simulink subsystem "Tire_Force"  (R2021b)
settings: Solver=VariableStepAuto  StartTime=0.0  StopTime=10.0  RelTol=1e-3
values from neighbouring files (symbols this model uses):
  afx_f = [1.736519934348130,-2.903281841026900e-04,2.651682004580759,7.000047010028531e+04,3.270011055825476e+03,-0.001252141095807,1.596836353939939]    [OneWheelModel_test1.m]    (also in OneWheelModel_test2.m)
  mu_tire_F = 0.55    [OneWheelModel_test1.m]    (also in OneWheelModel_test2.m)
libraries: simulink x1
settings Model: Creator=tsuyoshi  LastModifiedBy=tsuyoshi

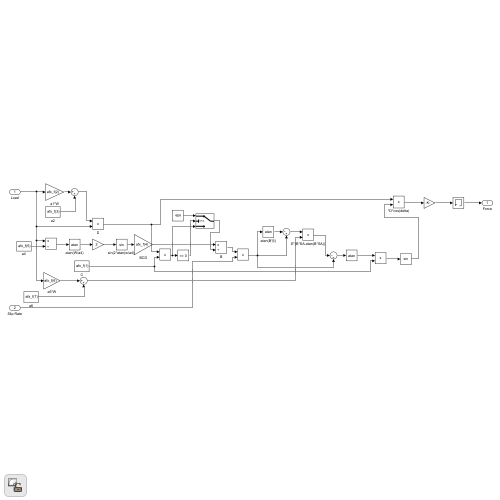
[thumbnail: Simulink's stored preview of the top-level diagram]
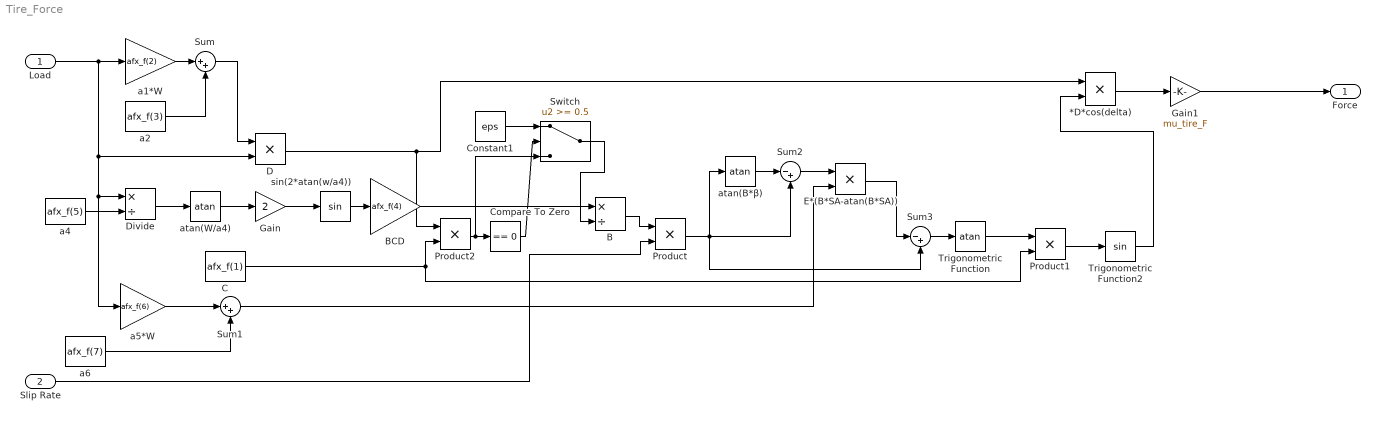
== system Tire_Force ==
  Load : Inport
  Slip Rate : Inport  Port=2
  *D*cos(delta) : Product  RndMeth=Zero
  B : Product  Inputs=*/
  BCD : Gain  Gain=afx_f(4)
  C : Constant  Value=afx_f(1)
  Compare To Zero : simulink/Logic and Bit Operations/Compare To Zero  relop===  OutDataTypeStr=boolean
  Constant1 : Constant  Value=eps
  D : Product  RndMeth=Zero
  Divide : Product  Inputs=*/
  E*(B*SA-atan(B*SA)) : Product  RndMeth=Zero
  Gain : Gain  Gain=2
  Gain1 : Gain  Gain=mu_tire_F
  Product : Product  RndMeth=Zero
  Product1 : Product  RndMeth=Zero
  Product2 : Product
  Sum : Sum  Inputs=|++
  Sum1 : Sum  Inputs=|++
  Sum2 : Sum  Inputs=|-+
  Sum3 : Sum  Inputs=|-+
  Switch : Switch  Threshold=0.5
  Trigonometric Function : Trigonometry  Operator=atan
  Trigonometric Function2 : Trigonometry
  a1*W : Gain  Gain=afx_f(2)
  a2 : Constant  Value=afx_f(3)
  a4 : Constant  Value=afx_f(5)
  a5*W : Gain  Gain=afx_f(6)
  a6 : Constant  Value=afx_f(7)
  atan(B*β) : Trigonometry  Operator=atan
  atan(W/a4) : Trigonometry  Operator=atan
  sin(2*atan(w/a4)) : Trigonometry
  Force : Outport  VectorParamsAs1DForOutWhenUnconnected=off
  wires:
  E*(B*SA-atan(B*SA))/1 -> Sum3/1
  Sum2/1 -> E*(B*SA-atan(B*SA))/1
  atan(B*β)/1 -> Sum2/1
  Product/1 -> Sum2/2, Sum3/2, atan(B*β)/1
  *D*cos(delta)/1 -> Gain1/1
  Switch/1 -> B/2
  Constant1/1 -> Switch/1
  Compare To Zero/1 -> Switch/2
  Product2/1 -> Switch/3, Compare To Zero/1
  Load/1 -> a5*W/1, Divide/1, D/2, a1*W/1
  Product1/1 -> Trigonometric Function2/1
  Trigonometric Function2/1 -> *D*cos(delta)/2
  Trigonometric Function/1 -> Product1/1
  D/1 -> Product2/1, *D*cos(delta)/1
  Sum3/1 -> Trigonometric Function/1
  Sum1/1 -> E*(B*SA-atan(B*SA))/2
  Slip Rate/1 -> Product/2
  B/1 -> Product/1
  a6/1 -> Sum1/2
  a5*W/1 -> Sum1/1
  C/1 -> Product1/2, Product2/2
  BCD/1 -> B/1
  sin(2*atan(w/a4))/1 -> BCD/1
  Gain/1 -> sin(2*atan(w/a4))/1
  atan(W/a4)/1 -> Gain/1
  Divide/1 -> atan(W/a4)/1
  a4/1 -> Divide/2
  Sum/1 -> D/1
  a1*W/1 -> Sum/1
  a2/1 -> Sum/2
  Gain1/1 -> Force/1
